simulink model "model"  (R2026a)
settings: Solver=VariableStepAuto
values from neighbouring files (symbols this model uses):
  Amg = 1    [data.m]
  B = 1    [data.m]
  J = 1    [data.m]
  Ls = 1    [data.m]
  p = 1    [data.m]
  Rs = 1    [data.m]

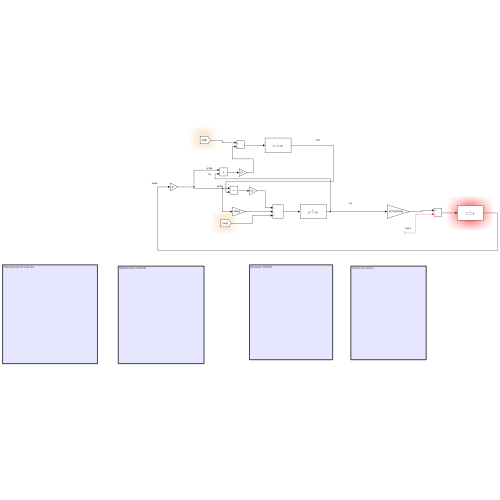
[thumbnail: Simulink's stored preview of the top-level diagram]
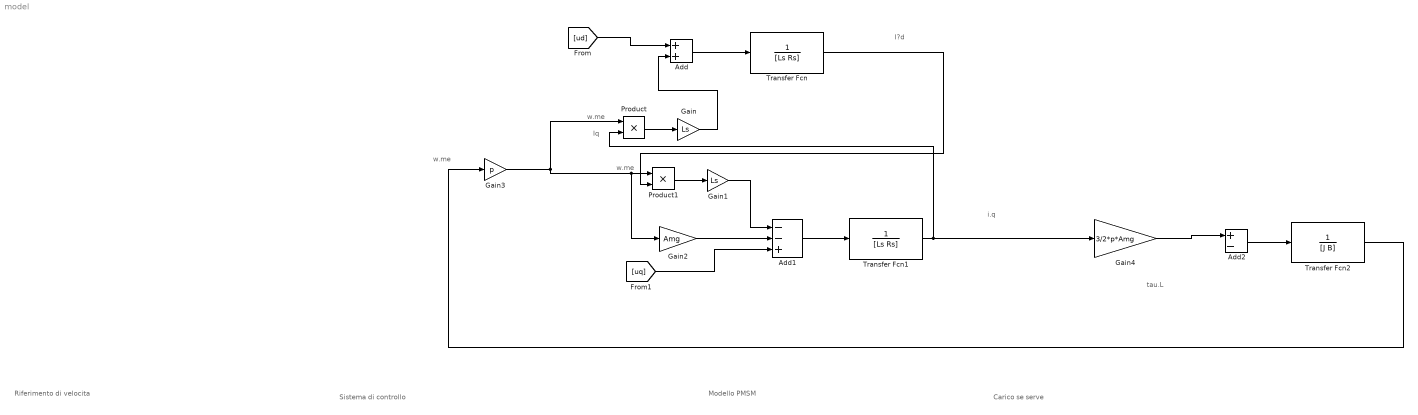
== system model ==
  note: tau.L
  note: w.me
  note: i.q
  note: I?d
  note: Iq
  note: w.me
  note: Carico se serve
  note: Riferimento di velocita
  note: Sistema di controllo
  note: Modello PMSM
  note: w.me
  Add : Sum
  Add1 : Sum  Inputs=--+
  Add2 : Sum  Inputs=+-
  Gain : Gain  Gain=Ls
  Gain1 : Gain  Gain=Ls
  Gain2 : Gain  Gain=Amg
  Gain3 : Gain  Gain=p
  Gain4 : Gain  Gain=3/2*p*Amg
  Product : Product
  Product1 : Product
  Transfer Fcn : TransferFcn  Denominator=[Ls Rs]
  Transfer Fcn1 : TransferFcn  Denominator=[Ls Rs]
  Transfer Fcn2 : TransferFcn  Denominator=[J B]
  wires:
  [ud] -> Add/1
  Product/1 -> Gain/1
  Gain/1 -> Add/2
  Add/1 -> Transfer Fcn/1
  Transfer Fcn/1 -> Product1/2
  Product1/1 -> Gain1/1
  Gain1/1 -> Add1/1
  Add1/1 -> Transfer Fcn1/1
  Transfer Fcn1/1 -> Product/2, Gain4/1
  [uq] -> Add1/3
  Gain2/1 -> Add1/2
  Gain3/1 -> Gain2/1, Product1/1, Product/1
  Transfer Fcn2/1 -> Gain3/1
  Gain4/1 -> Add2/1
  ? -> Add2/2
  Add2/1 -> Transfer Fcn2/1
